simulink model "LightControl"  (R2018a)
settings: configuration reference "ConfigSet" (kept outside this file)
values from neighbouring files (symbols this model uses):
  en_TurnSignal = <binary blob, 572 chars, not shown>    [CANLights.sldd]
  SteeringWheelPositionThresholdOff = 15.0    [CANLights.sldd]    (also in CANLights_dd2.sldd = 15.0)
  SteeringWheelPositionThresholdOn = 25.0    [CANLights.sldd]    (also in CANLights_dd2.sldd = 25.0)
libraries: simulink x3, dspswit3 x1
settings Model: DataDictionary=CANLights.sldd  ModifiedComment=jonathancoulter -- Thu Mar 15 17:11:06 2018 -- Version 1.7  ExtModeTrigDuration=2  Creator=Jonathan Coulter  LastModifiedBy=jonathancoulter
settings Model: ModifiedHistory=|
  | jonathancoulter -- Thu Mar 15 17:10:01 2018 -- Version 1.6
  | Initial model

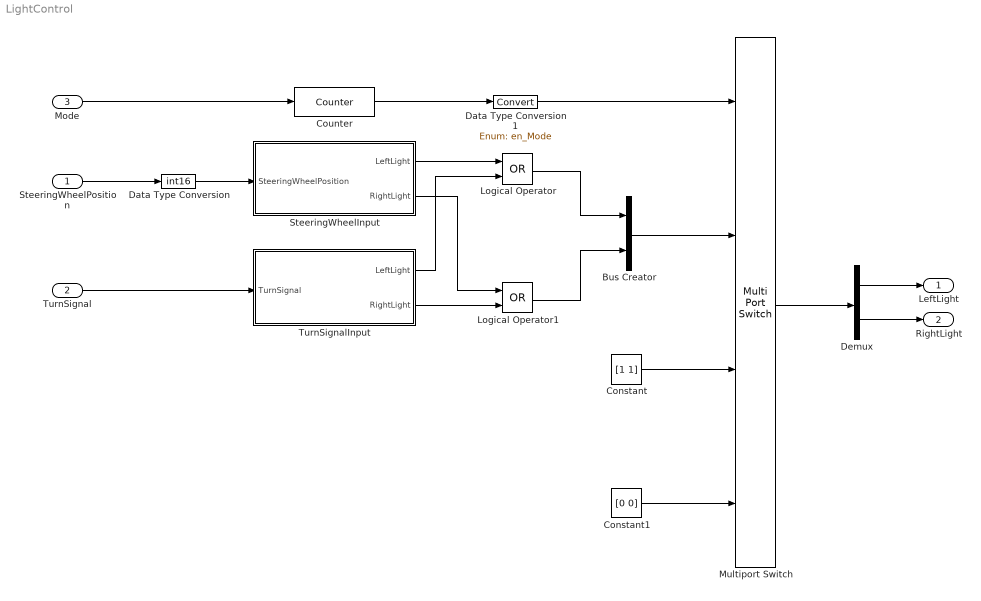
== system LightControl ==
  SteeringWheelPosition : Inport  OutDataTypeStr=dt_SteeringWheel
  TurnSignal : Inport  Port=2  OutDataTypeStr=Enum: en_TurnSignal
  Mode : Inport  Port=3  OutDataTypeStr=uint16
  Bus Creator : BusCreator  Inputs=2
  Constant : Constant  Value=[1 1]  OutDataTypeStr=boolean
  Constant1 : Constant  Value=[0 0]  OutDataTypeStr=boolean
  Counter : dspswit3/Counter  Direction=Up  CountEvent=Rising edge  CounterSize=User defined  MaxCount=2  InitialCount=0  Output=Count  HitValue=32  ResetInput=off  SamplesPerFrame=1  Ts=1  CntDtype=uint8  HitDtype=Logical
  Data Type Conversion : DataTypeConversion  OutDataTypeStr=int16
  Data Type Conversion1 : DataTypeConversion  OutDataTypeStr=Enum: en_Mode
  Demux : Demux  Outputs=2
  Logical Operator : Logic  Operator=OR  AllPortsSameDT=off  OutDataTypeStr=boolean
  Logical Operator1 : Logic  Operator=OR  AllPortsSameDT=off  OutDataTypeStr=boolean
  Multiport Switch : MultiPortSwitch  DataPortOrder=Specify indices  DataPortIndices={en_Mode.Auto, en_Mode.On, en_Mode.Off}  DiagnosticForDefault=None
  SteeringWheelInput : Subsystem
  TurnSignalInput : Subsystem
  LeftLight : Outport
  RightLight : Outport  Port=2
  wires:
  SteeringWheelPosition/1 -> Data Type Conversion/1
  TurnSignal/1 -> TurnSignalInput/1(TurnSignal)
  SteeringWheelInput/1(LeftLight) -> Logical Operator/1
  TurnSignalInput/1(LeftLight) -> Logical Operator/2
  SteeringWheelInput/2(RightLight) -> Logical Operator1/1
  TurnSignalInput/2(RightLight) -> Logical Operator1/2
  Data Type Conversion/1 -> SteeringWheelInput/1(SteeringWheelPosition)
  Mode/1 -> Counter/1
  Logical Operator/1 -> Bus Creator/1
  Logical Operator1/1 -> Bus Creator/2
  Counter/1 -> Data Type Conversion1/1
  Data Type Conversion1/1 -> Multiport Switch/1
  Bus Creator/1 -> Multiport Switch/2
  Constant/1 -> Multiport Switch/3
  Constant1/1 -> Multiport Switch/4
  Multiport Switch/1 -> Demux/1
  Demux/1 -> LeftLight/1
  Demux/2 -> RightLight/1

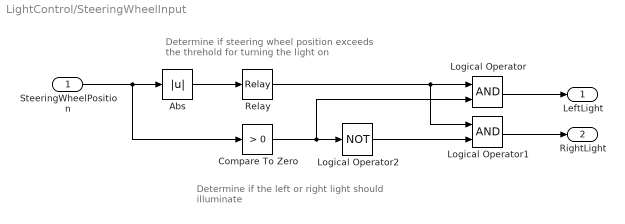
== system LightControl/SteeringWheelInput ==
  note: Determine if steering wheel position
      | exceeds the threhold for turning the light on
  note: Determine if the left or right light should
      | illuminate
  SteeringWheelPosition : Inport
  Abs : Abs  OutDataTypeStr=Inherit: Inherit via back propagation  SaturateOnIntegerOverflow=on
  Compare To Zero : simulink/Logic and Bit Operations/Compare To Zero  relop=>  OutDataTypeStr=boolean
  Logical Operator : Logic  AllPortsSameDT=off  OutDataTypeStr=boolean
  Logical Operator1 : Logic  AllPortsSameDT=off  OutDataTypeStr=boolean
  Logical Operator2 : Logic  Operator=NOT  AllPortsSameDT=off  OutDataTypeStr=boolean
  Relay : Relay  OnSwitchValue=SteeringWheelPositionThresholdOn  OffSwitchValue=SteeringWheelPositionThresholdOff  OutDataTypeStr=boolean
  LeftLight : Outport
  RightLight : Outport  Port=2
  wires:
  SteeringWheelPosition/1 -> Abs/1, Compare To Zero/1
  Abs/1 -> Relay/1
  Relay/1 -> Logical Operator1/1, Logical Operator/1
  Compare To Zero/1 -> Logical Operator2/1, Logical Operator/2
  Logical Operator/1 -> LeftLight/1
  Logical Operator1/1 -> RightLight/1
  Logical Operator2/1 -> Logical Operator1/2

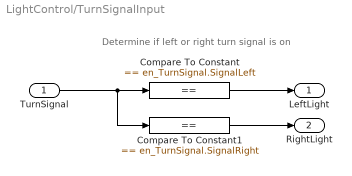
== system LightControl/TurnSignalInput ==
  note: Determine if left or right turn signal is on
  TurnSignal : Inport
  Compare To Constant : simulink/Logic and Bit Operations/Compare To Constant  relop===  const=en_TurnSignal.SignalLeft  OutDataTypeStr=boolean
  Compare To Constant1 : simulink/Logic and Bit Operations/Compare To Constant  relop===  const=en_TurnSignal.SignalRight  OutDataTypeStr=boolean
  LeftLight : Outport
  RightLight : Outport  Port=2
  wires:
  Compare To Constant/1 -> LeftLight/1
  TurnSignal/1 -> Compare To Constant1/1, Compare To Constant/1
  Compare To Constant1/1 -> RightLight/1
